simulink model "FullCardioLablModel"  (R2023b)
settings: Solver=FixedStepDiscrete  StartTime=0.0  StopTime=param_sim_time  FixedStep=1/fs  MaxStep=1/fs  RelTol=1e-3
undefined symbols (not defined in the file): analyses, fdesignblkfcn, fs, gcbh, param_tot_samples
libraries: dspstat3 x13, SCGAnalysis_SignalGenerationLib x2
(part 5 of 20)

== system FullCardioLablModel/ECG Preprocessing/Enabled ECG Preprocessing Subsystem/To Workspace: Processed ECG/Enabled To Workspace ECG Subsystem ==
  note: The subsystem is only enabled when it receives a (non-zero) signal
  In1 : Inport
  Enable : EnablePort
  To Workspace ECG : ToWorkspace  VariableName=out_ecg_preprocessing  SaveFormat=Structure  SampleTime=-1
  wires:
  In1/1 -> To Workspace ECG/1

== system FullCardioLablModel/SCG Analysis/Enabled SCG Analysis Subsystem/3D Anisotropy Characterization/Average Cycle Max Diameter//Volume Calculator ==
  in_r_pos : Inport
  in_scg_xyz : Inport  Port=2
  S1 Selector : Selector  NumberOfDimensions=2  InputPortWidth=3  IndexOptions=Index vector (dialog),Index vector (dialog)  Indices=[1:fs*0.2],[1 2 3]  OutputSizes=1,1
  SCG xyz Average Cycle : Subsystem
  Wrapped Average Cycle Max Diameter/Volume Calculator : MATLAB Function  TreatAsAtomicUnit=on
  out_average_cycle_max_diameter/volume : Outport
  wires:
  Wrapped Average Cycle Max Diameter/Volume Calculator/1(avg_cycle_max_diameter_over_volume) -> out_average_cycle_max_diameter/volume/1
  SCG xyz Average Cycle/1(out_scg_xyz_avgcycle) -> S1 Selector/1
  in_scg_xyz/1 -> SCG xyz Average Cycle/2(in_scg_xyz)
  in_r_pos/1 -> SCG xyz Average Cycle/1(in_ecg_r)
  S1 Selector/1 -> Wrapped Average Cycle Max Diameter/Volume Calculator/1(avg_s1_xyz)  "avg_scg_xyz_s1"

== system FullCardioLablModel/SCG Analysis/Enabled SCG Analysis Subsystem/3D Anisotropy Characterization/Average Cycle Max//Median Diameter Calculator ==
  in_r_pos : Inport
  in_scg_xyz : Inport  Port=2
  S1 Selector : Selector  NumberOfDimensions=2  InputPortWidth=3  IndexOptions=Index vector (dialog),Index vector (dialog)  Indices=[1:fs*0.2],[1 2 3]  OutputSizes=1,1
  SCG xyz Average Cycle : Subsystem
  Wrapped Average Cycle Max/Median Diameter Calculator : MATLAB Function  TreatAsAtomicUnit=on
  out_average_cycle_max/median_diameter : Outport
  wires:
  Wrapped Average Cycle Max/Median Diameter Calculator/1(avg_cycle_max_over_median_diameter) -> out_average_cycle_max/median_diameter/1
  SCG xyz Average Cycle/1(out_scg_xyz_avgcycle) -> S1 Selector/1
  in_scg_xyz/1 -> SCG xyz Average Cycle/2(in_scg_xyz)
  in_r_pos/1 -> SCG xyz Average Cycle/1(in_ecg_r)
  S1 Selector/1 -> Wrapped Average Cycle Max/Median Diameter Calculator/1(avg_s1_xyz)  "avg_scg_xyz_s1"

== system FullCardioLablModel/SCG Analysis/Enabled SCG Analysis Subsystem/3D Anisotropy Characterization/Average Cycle Max//Min Diameter Calculator ==
  in_r_pos : Inport
  in_scg_xyz : Inport  Port=2
  S1 Selector : Selector  NumberOfDimensions=2  InputPortWidth=3  IndexOptions=Index vector (dialog),Index vector (dialog)  Indices=[1:fs*0.2],[1 2 3]  OutputSizes=1,1
  SCG xyz Average Cycle : Subsystem
  Wrapped Average Cycle Max/Min Diameters Calculator : MATLAB Function  TreatAsAtomicUnit=on
  out_average_cycle_max/min_diameter : Outport
  wires:
  S1 Selector/1 -> Wrapped Average Cycle Max/Min Diameters Calculator/1(avg_s1_xyz)  "avg_scg_xyz_s1"
  in_r_pos/1 -> SCG xyz Average Cycle/1(in_ecg_r)
  in_scg_xyz/1 -> SCG xyz Average Cycle/2(in_scg_xyz)
  SCG xyz Average Cycle/1(out_scg_xyz_avgcycle) -> S1 Selector/1
  Wrapped Average Cycle Max/Min Diameters Calculator/1(avg_cycle_max_over_min_diameters) -> out_average_cycle_max/min_diameter/1

== system FullCardioLablModel/SCG Analysis/Enabled SCG Analysis Subsystem/3D Anisotropy Characterization/Average Max Diameter//Volume Calculator ==
  in_r_pos : Inport
  in_scg_xyz : Inport  Port=2
  Constant1 : Constant  Value=fs
  Wrapped Average Max Diameter/Volume Calculator : MATLAB Function  TreatAsAtomicUnit=on
  out_average_max_diameter/volume : Outport
  wires:
  Constant1/1 -> Wrapped Average Max Diameter/Volume Calculator/1(fs)
  Wrapped Average Max Diameter/Volume Calculator/1(avg_max_diameter_over_volume) -> out_average_max_diameter/volume/1
  in_scg_xyz/1 -> Wrapped Average Max Diameter/Volume Calculator/3(scg_xyz)
  in_r_pos/1 -> Wrapped Average Max Diameter/Volume Calculator/2(r_pos)

== system FullCardioLablModel/SCG Analysis/Enabled SCG Analysis Subsystem/3D Anisotropy Characterization/Average Max//Median Diameter Calculator ==
  in_r_pos : Inport
  in_scg_xyz : Inport  Port=2
  Constant1 : Constant  Value=fs
  Wrapped Average Max/Median Diameter Calculator : MATLAB Function  TreatAsAtomicUnit=on
  out_average_max/median_diameter : Outport
  wires:
  Constant1/1 -> Wrapped Average Max/Median Diameter Calculator/1(fs)
  Wrapped Average Max/Median Diameter Calculator/1(avg_max_over_median_diameter) -> out_average_max/median_diameter/1
  in_scg_xyz/1 -> Wrapped Average Max/Median Diameter Calculator/3(scg_xyz)
  in_r_pos/1 -> Wrapped Average Max/Median Diameter Calculator/2(r_pos)

== system FullCardioLablModel/SCG Analysis/Enabled SCG Analysis Subsystem/3D Anisotropy Characterization/Average Max//Min Diameter Calculator ==
  in_r_pos : Inport
  in_scg_xyz : Inport  Port=2
  Constant1 : Constant  Value=fs
  Wrapped Average Max/Min Diameters Calculator : MATLAB Function  TreatAsAtomicUnit=on
  out_average_max/min_diameter : Outport
  wires:
  in_r_pos/1 -> Wrapped Average Max/Min Diameters Calculator/2(r_pos)
  in_scg_xyz/1 -> Wrapped Average Max/Min Diameters Calculator/3(scg_xyz)
  Wrapped Average Max/Min Diameters Calculator/1(avg_max_over_min_diameters) -> out_average_max/min_diameter/1
  Constant1/1 -> Wrapped Average Max/Min Diameters Calculator/1(fs)

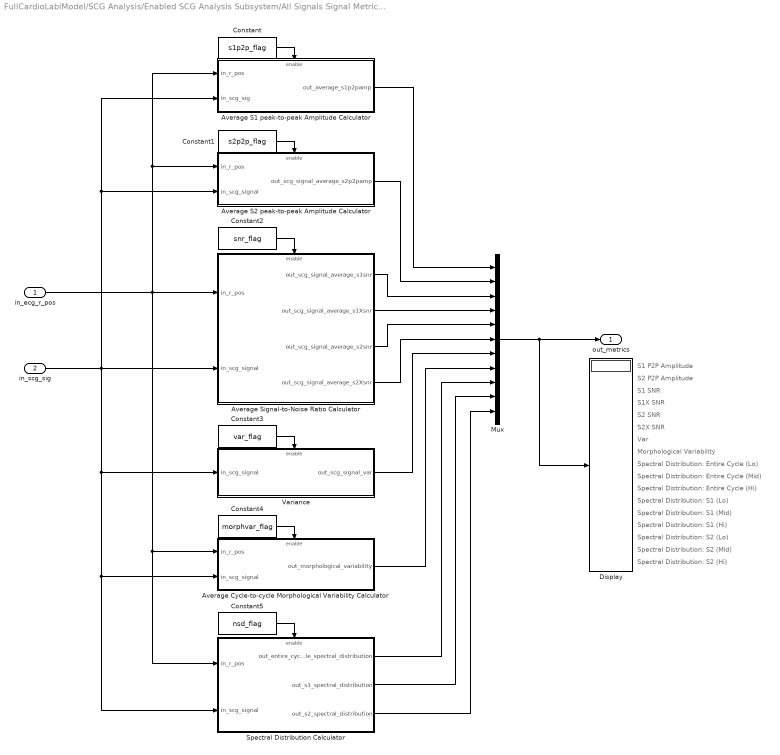
== system FullCardioLablModel/SCG Analysis/Enabled SCG Analysis Subsystem/All Signals Signal Metric Characterization/SCG 2D Mod Signal Metric Characterization ==
  note: S1 P2P Amplitude
  note: S2 P2P Amplitude
  note: S1 SNR
  note: S1X SNR
  note: S2 SNR
  note: S2X SNR
  note: Var
  note: Morphological Variability
  note: Spectral Distribution: Entire Cycle (Lo)
  note: Spectral Distribution: Entire Cycle (Mid)
  note: Spectral Distribution: Entire Cycle (Hi)
  note: Spectral Distribution: S1 (Lo)
  note: Spectral Distribution: S1 (Mid)
  note: Spectral Distribution: S1 (Hi)
  note: Spectral Distribution: S2 (Hi)
  note: Spectral Distribution: S2 (Lo)
  note: Spectral Distribution: S2 (Mid)
  in_ecg_r_pos : Inport
  in_scg_sig : Inport  Port=2
  Average Cycle-to-cycle Morphological Variability Calculator : Subsystem
  Average S1 peak-to-peak Amplitude Calculator : Subsystem
  Average S2 peak-to-peak Amplitude Calculator : Subsystem
  Average Signal-to-Noise Ratio Calculator : Subsystem  mask{s1snr_flag=on, s1xsnr_flag=on, s2snr_flag=on, s2xsnr_flag=on}
      mask prompts: s1snr_flag "S1 SnR"; s1xsnr_flag "S1X SnR (S2 complex is removed)"; s2snr_flag "S2 SnR"; s2xsnr_flag "S2X SnR (S1 complex is removed)"
      mask DialogControl DescGroupVar Prompt: Signal-to-Noise Ratio Characterization
      mask DialogControl DescTextVar Prompt: Block to quantify the signal to noise ratio of the S1 and S2 complexes. Two types of SnRs can be calculated: the normal SnR (which reflects the ease of performing an independent detection of that complex), and the exclusive SnR (which does not cosider the S2 or S1 complex in the case of the S1 and S2 SnRs, respectively).
      mask DialogControl Control2 Prompt: Choose which SnRs to compute:
  Constant : Constant  Value=s1p2p_flag
  Constant1 : Constant  Value=s2p2p_flag
  Constant2 : Constant  Value=snr_flag
  Constant3 : Constant  Value=var_flag
  Constant4 : Constant  Value=morphvar_flag
  Constant5 : Constant  Value=nsd_flag
  Display : Display
  Mux : Mux  Inputs=11
  Spectral Distribution Calculator : Subsystem  mask{entire_cycle=on, s1=on, s2=on, f_band_lo=[7.5 15], f_band_mid=[15 30], f_band_hi=[30 120]}
      mask prompts: entire_cycle "Entire Cycle"; s1 "S1 Complex"; s2 "S2 Complex"; f_band_lo "Frequency Band Low Limits (Hz)"; f_band_mid "Frequency Band Mid Limits (Hz)"; f_band_hi "Frequency Band Hi Limits (Hz)"
      mask DialogControl DescGroupVar Prompt: Spectral Distribution Calculator
      mask DialogControl DescTextVar Prompt: Block to calculate the (normalized) distrubtions of the power spectral densities of: the entire cycle, the S1 complex, and the S2 complex. First select which combination of spectral distrubtions to calculate. Then enter the frequency limits (in Hz) of the three contiguos bins that will define the spectral distribution.
      mask DialogControl ParameterGroupVar_copy Prompt: Spectral Distributions to Calculate
      mask DialogControl Control4 Prompt: Select which spectral distributions to calculate.
      mask DialogControl ParameterGroupVar Prompt: Bin Frequency Bands
      mask DialogControl Control2 Prompt: Enter the frequency limits (in Hz) inside square brackets for three contiguous bins (e.g. [5 10], [10 40], and [40 120]).
  Variance : Subsystem
  out_metrics : Outport
  wires:
  in_scg_sig/1 -> Average S2 peak-to-peak Amplitude Calculator/2(in_scg_signal), Average S1 peak-to-peak Amplitude Calculator/2(in_scg_sig), Average Signal-to-Noise Ratio Calculator/2(in_scg_signal), Spectral Distribution Calculator/2(in_scg_signal), Average Cycle-to-cycle Morphological Variability Calculator/2(in_scg_signal), Variance/1(in_scg_signal)
  Average S1 peak-to-peak Amplitude Calculator/1(out_average_s1p2pamp) -> Mux/1
  in_ecg_r_pos/1 -> Spectral Distribution Calculator/1(in_r_pos), Average Cycle-to-cycle Morphological Variability Calculator/1(in_r_pos), Average S2 peak-to-peak Amplitude Calculator/1(in_r_pos), Average S1 peak-to-peak Amplitude Calculator/1(in_r_pos), Average Signal-to-Noise Ratio Calculator/1(in_r_pos)
  Average Signal-to-Noise Ratio Calculator/2(out_scg_signal_average_s1Xsnr) -> Mux/4
  Average Signal-to-Noise Ratio Calculator/1(out_scg_signal_average_s1snr) -> Mux/3
  Average Signal-to-Noise Ratio Calculator/3(out_scg_signal_average_s2snr) -> Mux/5
  Average Signal-to-Noise Ratio Calculator/4(out_scg_signal_average_s2Xsnr) -> Mux/6
  Average S2 peak-to-peak Amplitude Calculator/1(out_scg_signal_average_s2p2pamp) -> Mux/2
  Average Cycle-to-cycle Morphological Variability Calculator/1(out_morphological_variability) -> Mux/8
  Spectral Distribution Calculator/1(out_entire_cycle_spectral_distribution) -> Mux/9
  Spectral Distribution Calculator/3(out_s2_spectral_distribution) -> Mux/11
  Spectral Distribution Calculator/2(out_s1_spectral_distribution) -> Mux/10
  Variance/1(out_scg_signal_var) -> Mux/7
  Constant/1 -> Average S1 peak-to-peak Amplitude Calculator/Enable
  Constant1/1 -> Average S2 peak-to-peak Amplitude Calculator/Enable
  Constant2/1 -> Average Signal-to-Noise Ratio Calculator/Enable
  Constant3/1 -> Variance/Enable
  Constant4/1 -> Average Cycle-to-cycle Morphological Variability Calculator/Enable
  Constant5/1 -> Spectral Distribution Calculator/Enable
  Mux/1 -> Display/1, out_metrics/1

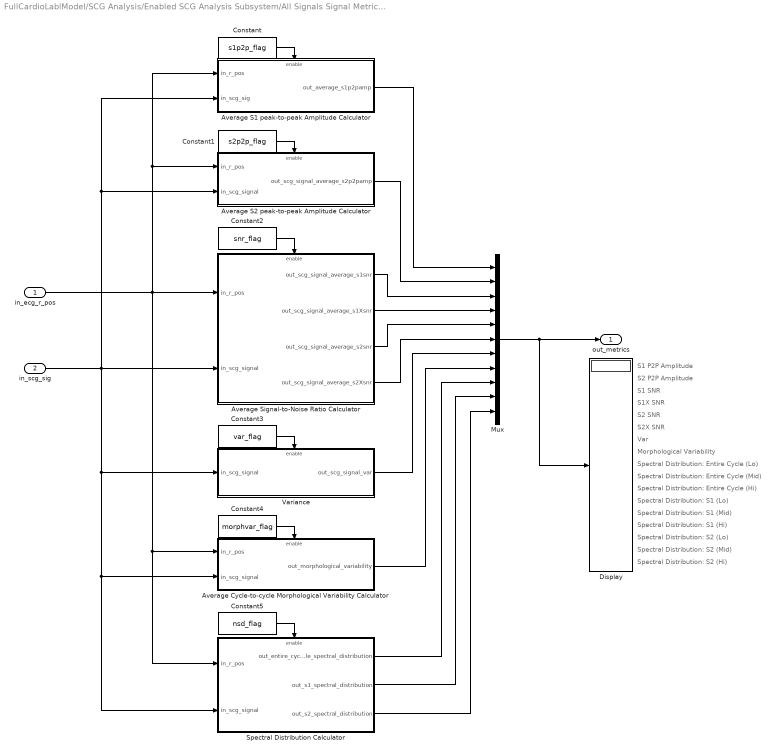
== system FullCardioLablModel/SCG Analysis/Enabled SCG Analysis Subsystem/All Signals Signal Metric Characterization/SCG 3D Mod Signal Metric Characterization ==
  note: Spectral Distribution: S2 (Mid)
  note: Spectral Distribution: S2 (Lo)
  note: Spectral Distribution: S2 (Hi)
  note: Spectral Distribution: S1 (Hi)
  note: Spectral Distribution: S1 (Mid)
  note: Spectral Distribution: S1 (Lo)
  note: Spectral Distribution: Entire Cycle (Hi)
  note: Spectral Distribution: Entire Cycle (Mid)
  note: Spectral Distribution: Entire Cycle (Lo)
  note: Morphological Variability
  note: Var
  note: S2X SNR
  note: S2 SNR
  note: S1X SNR
  note: S1 SNR
  note: S2 P2P Amplitude
  note: S1 P2P Amplitude
  in_ecg_r_pos : Inport
  in_scg_sig : Inport  Port=2
  Average Cycle-to-cycle Morphological Variability Calculator : Subsystem
  Average S1 peak-to-peak Amplitude Calculator : Subsystem
  Average S2 peak-to-peak Amplitude Calculator : Subsystem
  Average Signal-to-Noise Ratio Calculator : Subsystem  mask{s1snr_flag=on, s1xsnr_flag=on, s2snr_flag=on, s2xsnr_flag=on}
      mask prompts: s1snr_flag "S1 SnR"; s1xsnr_flag "S1X SnR (S2 complex is removed)"; s2snr_flag "S2 SnR"; s2xsnr_flag "S2X SnR (S1 complex is removed)"
      mask DialogControl DescGroupVar Prompt: Signal-to-Noise Ratio Characterization
      mask DialogControl DescTextVar Prompt: Block to quantify the signal to noise ratio of the S1 and S2 complexes. Two types of SnRs can be calculated: the normal SnR (which reflects the ease of performing an independent detection of that complex), and the exclusive SnR (which does not cosider the S2 or S1 complex in the case of the S1 and S2 SnRs, respectively).
      mask DialogControl Control2 Prompt: Choose which SnRs to compute:
  Constant : Constant  Value=s1p2p_flag
  Constant1 : Constant  Value=s2p2p_flag
  Constant2 : Constant  Value=snr_flag
  Constant3 : Constant  Value=var_flag
  Constant4 : Constant  Value=morphvar_flag
  Constant5 : Constant  Value=nsd_flag
  Display : Display
  Mux : Mux  Inputs=11
  Spectral Distribution Calculator : Subsystem  mask{entire_cycle=on, s1=on, s2=on, f_band_lo=[7.5 15], f_band_mid=[15 30], f_band_hi=[30 120]}
      mask prompts: entire_cycle "Entire Cycle"; s1 "S1 Complex"; s2 "S2 Complex"; f_band_lo "Frequency Band Low Limits (Hz)"; f_band_mid "Frequency Band Mid Limits (Hz)"; f_band_hi "Frequency Band Hi Limits (Hz)"
      mask DialogControl DescGroupVar Prompt: Spectral Distribution Calculator
      mask DialogControl DescTextVar Prompt: Block to calculate the (normalized) distrubtions of the power spectral densities of: the entire cycle, the S1 complex, and the S2 complex. First select which combination of spectral distrubtions to calculate. Then enter the frequency limits (in Hz) of the three contiguos bins that will define the spectral distribution.
      mask DialogControl ParameterGroupVar_copy Prompt: Spectral Distributions to Calculate
      mask DialogControl Control4 Prompt: Select which spectral distributions to calculate.
      mask DialogControl ParameterGroupVar Prompt: Bin Frequency Bands
      mask DialogControl Control2 Prompt: Enter the frequency limits (in Hz) inside square brackets for three contiguous bins (e.g. [5 10], [10 40], and [40 120]).
  Variance : Subsystem
  out_metrics : Outport
  wires:
  Mux/1 -> out_metrics/1, Display/1
  Constant5/1 -> Spectral Distribution Calculator/Enable
  Constant4/1 -> Average Cycle-to-cycle Morphological Variability Calculator/Enable
  Constant3/1 -> Variance/Enable
  Constant2/1 -> Average Signal-to-Noise Ratio Calculator/Enable
  Constant1/1 -> Average S2 peak-to-peak Amplitude Calculator/Enable
  Constant/1 -> Average S1 peak-to-peak Amplitude Calculator/Enable
  Variance/1(out_scg_signal_var) -> Mux/7
  Spectral Distribution Calculator/2(out_s1_spectral_distribution) -> Mux/10
  Spectral Distribution Calculator/3(out_s2_spectral_distribution) -> Mux/11
  Spectral Distribution Calculator/1(out_entire_cycle_spectral_distribution) -> Mux/9
  Average Cycle-to-cycle Morphological Variability Calculator/1(out_morphological_variability) -> Mux/8
  Average S2 peak-to-peak Amplitude Calculator/1(out_scg_signal_average_s2p2pamp) -> Mux/2
  Average Signal-to-Noise Ratio Calculator/4(out_scg_signal_average_s2Xsnr) -> Mux/6
  Average Signal-to-Noise Ratio Calculator/3(out_scg_signal_average_s2snr) -> Mux/5
  Average Signal-to-Noise Ratio Calculator/1(out_scg_signal_average_s1snr) -> Mux/3
  Average Signal-to-Noise Ratio Calculator/2(out_scg_signal_average_s1Xsnr) -> Mux/4
  in_ecg_r_pos/1 -> Average Signal-to-Noise Ratio Calculator/1(in_r_pos), Average S1 peak-to-peak Amplitude Calculator/1(in_r_pos), Average S2 peak-to-peak Amplitude Calculator/1(in_r_pos), Average Cycle-to-cycle Morphological Variability Calculator/1(in_r_pos), Spectral Distribution Calculator/1(in_r_pos)
  Average S1 peak-to-peak Amplitude Calculator/1(out_average_s1p2pamp) -> Mux/1
  in_scg_sig/1 -> Average S1 peak-to-peak Amplitude Calculator/2(in_scg_sig), Average S2 peak-to-peak Amplitude Calculator/2(in_scg_signal), Average Signal-to-Noise Ratio Calculator/2(in_scg_signal), Variance/1(in_scg_signal), Average Cycle-to-cycle Morphological Variability Calculator/2(in_scg_signal), Spectral Distribution Calculator/2(in_scg_signal)

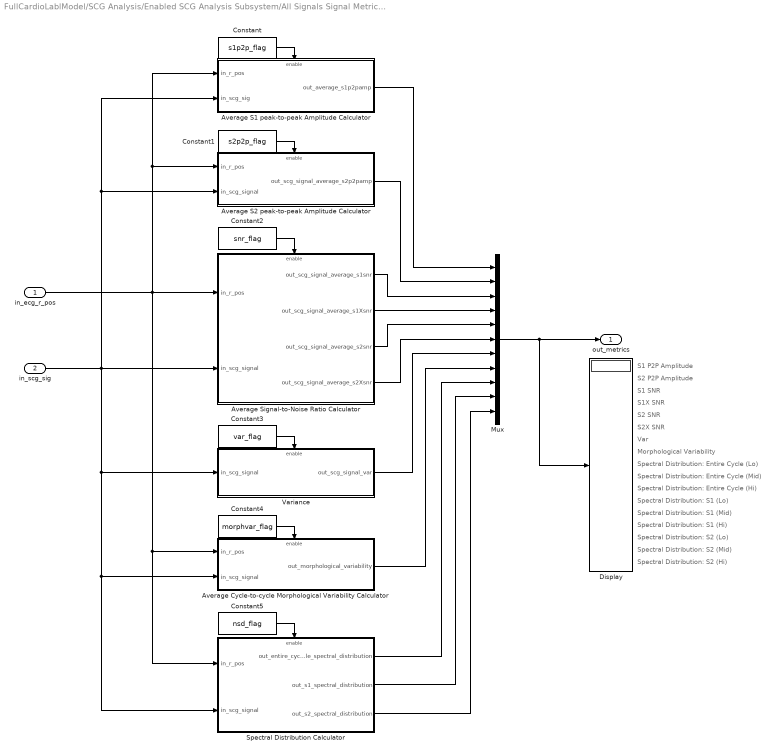
== system FullCardioLablModel/SCG Analysis/Enabled SCG Analysis Subsystem/All Signals Signal Metric Characterization/SCG 3DMaxS2p2pProjection Signal Metric Characterization ==
  note: Spectral Distribution: S2 (Mid)
  note: Spectral Distribution: S2 (Lo)
  note: Spectral Distribution: S2 (Hi)
  note: Spectral Distribution: S1 (Hi)
  note: Spectral Distribution: S1 (Mid)
  note: Spectral Distribution: S1 (Lo)
  note: Spectral Distribution: Entire Cycle (Hi)
  note: Spectral Distribution: Entire Cycle (Mid)
  note: Spectral Distribution: Entire Cycle (Lo)
  note: Morphological Variability
  note: Var
  note: S2X SNR
  note: S2 SNR
  note: S1X SNR
  note: S1 SNR
  note: S2 P2P Amplitude
  note: S1 P2P Amplitude
  in_ecg_r_pos : Inport
  in_scg_sig : Inport  Port=2
  Average Cycle-to-cycle Morphological Variability Calculator : Subsystem
  Average S1 peak-to-peak Amplitude Calculator : Subsystem
  Average S2 peak-to-peak Amplitude Calculator : Subsystem
  Average Signal-to-Noise Ratio Calculator : Subsystem  mask{s1snr_flag=on, s1xsnr_flag=on, s2snr_flag=on, s2xsnr_flag=on}
      mask prompts: s1snr_flag "S1 SnR"; s1xsnr_flag "S1X SnR (S2 complex is removed)"; s2snr_flag "S2 SnR"; s2xsnr_flag "S2X SnR (S1 complex is removed)"
      mask DialogControl DescGroupVar Prompt: Signal-to-Noise Ratio Characterization
      mask DialogControl DescTextVar Prompt: Block to quantify the signal to noise ratio of the S1 and S2 complexes. Two types of SnRs can be calculated: the normal SnR (which reflects the ease of performing an independent detection of that complex), and the exclusive SnR (which does not cosider the S2 or S1 complex in the case of the S1 and S2 SnRs, respectively).
      mask DialogControl Control2 Prompt: Choose which SnRs to compute:
  Constant : Constant  Value=s1p2p_flag
  Constant1 : Constant  Value=s2p2p_flag
  Constant2 : Constant  Value=snr_flag
  Constant3 : Constant  Value=var_flag
  Constant4 : Constant  Value=morphvar_flag
  Constant5 : Constant  Value=nsd_flag
  Display : Display
  Mux : Mux  Inputs=11
  Spectral Distribution Calculator : Subsystem  mask{entire_cycle=on, s1=on, s2=on, f_band_lo=[7.5 15], f_band_mid=[15 30], f_band_hi=[30 120]}
      mask prompts: entire_cycle "Entire Cycle"; s1 "S1 Complex"; s2 "S2 Complex"; f_band_lo "Frequency Band Low Limits (Hz)"; f_band_mid "Frequency Band Mid Limits (Hz)"; f_band_hi "Frequency Band Hi Limits (Hz)"
      mask DialogControl DescGroupVar Prompt: Spectral Distribution Calculator
      mask DialogControl DescTextVar Prompt: Block to calculate the (normalized) distrubtions of the power spectral densities of: the entire cycle, the S1 complex, and the S2 complex. First select which combination of spectral distrubtions to calculate. Then enter the frequency limits (in Hz) of the three contiguos bins that will define the spectral distribution.
      mask DialogControl ParameterGroupVar_copy Prompt: Spectral Distributions to Calculate
      mask DialogControl Control4 Prompt: Select which spectral distributions to calculate.
      mask DialogControl ParameterGroupVar Prompt: Bin Frequency Bands
      mask DialogControl Control2 Prompt: Enter the frequency limits (in Hz) inside square brackets for three contiguous bins (e.g. [5 10], [10 40], and [40 120]).
  Variance : Subsystem
  out_metrics : Outport
  wires:
  Mux/1 -> out_metrics/1, Display/1
  Constant5/1 -> Spectral Distribution Calculator/Enable
  Constant4/1 -> Average Cycle-to-cycle Morphological Variability Calculator/Enable
  Constant3/1 -> Variance/Enable
  Constant2/1 -> Average Signal-to-Noise Ratio Calculator/Enable
  Constant1/1 -> Average S2 peak-to-peak Amplitude Calculator/Enable
  Constant/1 -> Average S1 peak-to-peak Amplitude Calculator/Enable
  Variance/1(out_scg_signal_var) -> Mux/7
  Spectral Distribution Calculator/2(out_s1_spectral_distribution) -> Mux/10
  Spectral Distribution Calculator/3(out_s2_spectral_distribution) -> Mux/11
  Spectral Distribution Calculator/1(out_entire_cycle_spectral_distribution) -> Mux/9
  Average Cycle-to-cycle Morphological Variability Calculator/1(out_morphological_variability) -> Mux/8
  Average S2 peak-to-peak Amplitude Calculator/1(out_scg_signal_average_s2p2pamp) -> Mux/2
  Average Signal-to-Noise Ratio Calculator/4(out_scg_signal_average_s2Xsnr) -> Mux/6
  Average Signal-to-Noise Ratio Calculator/3(out_scg_signal_average_s2snr) -> Mux/5
  Average Signal-to-Noise Ratio Calculator/1(out_scg_signal_average_s1snr) -> Mux/3
  Average Signal-to-Noise Ratio Calculator/2(out_scg_signal_average_s1Xsnr) -> Mux/4
  in_ecg_r_pos/1 -> Average Signal-to-Noise Ratio Calculator/1(in_r_pos), Average S1 peak-to-peak Amplitude Calculator/1(in_r_pos), Average S2 peak-to-peak Amplitude Calculator/1(in_r_pos), Average Cycle-to-cycle Morphological Variability Calculator/1(in_r_pos), Spectral Distribution Calculator/1(in_r_pos)
  Average S1 peak-to-peak Amplitude Calculator/1(out_average_s1p2pamp) -> Mux/1
  in_scg_sig/1 -> Average S1 peak-to-peak Amplitude Calculator/2(in_scg_sig), Average S2 peak-to-peak Amplitude Calculator/2(in_scg_signal), Average Signal-to-Noise Ratio Calculator/2(in_scg_signal), Variance/1(in_scg_signal), Average Cycle-to-cycle Morphological Variability Calculator/2(in_scg_signal), Spectral Distribution Calculator/2(in_scg_signal)

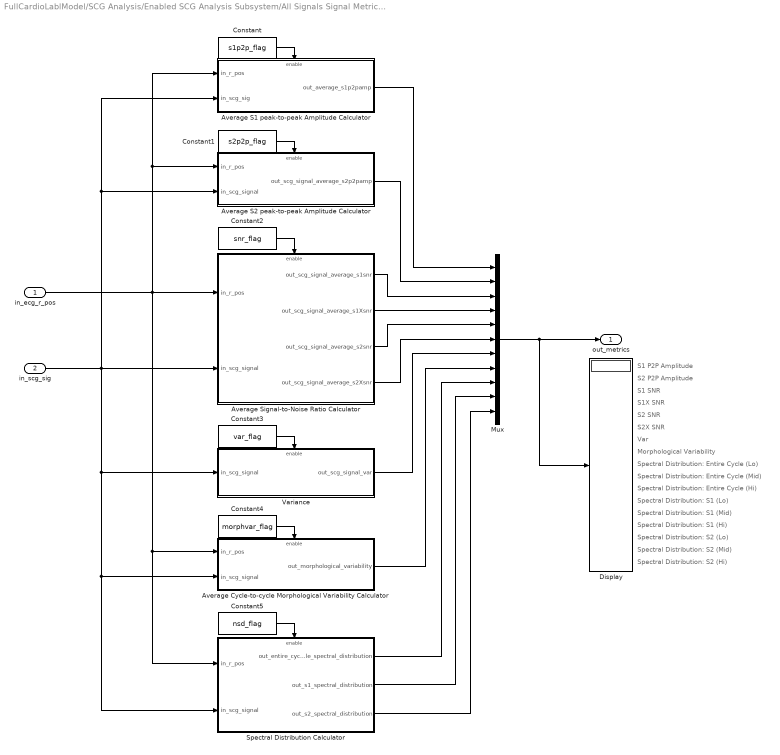
== system FullCardioLablModel/SCG Analysis/Enabled SCG Analysis Subsystem/All Signals Signal Metric Characterization/SCG 3DMinS2p2pProjection Signal Metric Characterization ==
  note: S1 P2P Amplitude
  note: S2 P2P Amplitude
  note: S1 SNR
  note: S1X SNR
  note: S2 SNR
  note: S2X SNR
  note: Var
  note: Morphological Variability
  note: Spectral Distribution: Entire Cycle (Lo)
  note: Spectral Distribution: Entire Cycle (Mid)
  note: Spectral Distribution: Entire Cycle (Hi)
  note: Spectral Distribution: S1 (Lo)
  note: Spectral Distribution: S1 (Mid)
  note: Spectral Distribution: S1 (Hi)
  note: Spectral Distribution: S2 (Hi)
  note: Spectral Distribution: S2 (Lo)
  note: Spectral Distribution: S2 (Mid)
  in_ecg_r_pos : Inport
  in_scg_sig : Inport  Port=2
  Average Cycle-to-cycle Morphological Variability Calculator : Subsystem
  Average S1 peak-to-peak Amplitude Calculator : Subsystem
  Average S2 peak-to-peak Amplitude Calculator : Subsystem
  Average Signal-to-Noise Ratio Calculator : Subsystem  mask{s1snr_flag=on, s1xsnr_flag=on, s2snr_flag=on, s2xsnr_flag=on}
      mask prompts: s1snr_flag "S1 SnR"; s1xsnr_flag "S1X SnR (S2 complex is removed)"; s2snr_flag "S2 SnR"; s2xsnr_flag "S2X SnR (S1 complex is removed)"
      mask DialogControl DescGroupVar Prompt: Signal-to-Noise Ratio Characterization
      mask DialogControl DescTextVar Prompt: Block to quantify the signal to noise ratio of the S1 and S2 complexes. Two types of SnRs can be calculated: the normal SnR (which reflects the ease of performing an independent detection of that complex), and the exclusive SnR (which does not cosider the S2 or S1 complex in the case of the S1 and S2 SnRs, respectively).
      mask DialogControl Control2 Prompt: Choose which SnRs to compute:
  Constant : Constant  Value=s1p2p_flag
  Constant1 : Constant  Value=s2p2p_flag
  Constant2 : Constant  Value=snr_flag
  Constant3 : Constant  Value=var_flag
  Constant4 : Constant  Value=morphvar_flag
  Constant5 : Constant  Value=nsd_flag
  Display : Display
  Mux : Mux  Inputs=11
  Spectral Distribution Calculator : Subsystem  mask{entire_cycle=on, s1=on, s2=on, f_band_lo=[7.5 15], f_band_mid=[15 30], f_band_hi=[30 120]}
      mask prompts: entire_cycle "Entire Cycle"; s1 "S1 Complex"; s2 "S2 Complex"; f_band_lo "Frequency Band Low Limits (Hz)"; f_band_mid "Frequency Band Mid Limits (Hz)"; f_band_hi "Frequency Band Hi Limits (Hz)"
      mask DialogControl DescGroupVar Prompt: Spectral Distribution Calculator
      mask DialogControl DescTextVar Prompt: Block to calculate the (normalized) distrubtions of the power spectral densities of: the entire cycle, the S1 complex, and the S2 complex. First select which combination of spectral distrubtions to calculate. Then enter the frequency limits (in Hz) of the three contiguos bins that will define the spectral distribution.
      mask DialogControl ParameterGroupVar_copy Prompt: Spectral Distributions to Calculate
      mask DialogControl Control4 Prompt: Select which spectral distributions to calculate.
      mask DialogControl ParameterGroupVar Prompt: Bin Frequency Bands
      mask DialogControl Control2 Prompt: Enter the frequency limits (in Hz) inside square brackets for three contiguous bins (e.g. [5 10], [10 40], and [40 120]).
  Variance : Subsystem
  out_metrics : Outport
  wires:
  in_scg_sig/1 -> Average S2 peak-to-peak Amplitude Calculator/2(in_scg_signal), Average S1 peak-to-peak Amplitude Calculator/2(in_scg_sig), Spectral Distribution Calculator/2(in_scg_signal), Average Cycle-to-cycle Morphological Variability Calculator/2(in_scg_signal), Variance/1(in_scg_signal), Average Signal-to-Noise Ratio Calculator/2(in_scg_signal)
  Average S1 peak-to-peak Amplitude Calculator/1(out_average_s1p2pamp) -> Mux/1
  in_ecg_r_pos/1 -> Spectral Distribution Calculator/1(in_r_pos), Average Cycle-to-cycle Morphological Variability Calculator/1(in_r_pos), Average S2 peak-to-peak Amplitude Calculator/1(in_r_pos), Average S1 peak-to-peak Amplitude Calculator/1(in_r_pos), Average Signal-to-Noise Ratio Calculator/1(in_r_pos)
  Average Signal-to-Noise Ratio Calculator/2(out_scg_signal_average_s1Xsnr) -> Mux/4
  Average Signal-to-Noise Ratio Calculator/1(out_scg_signal_average_s1snr) -> Mux/3
  Average Signal-to-Noise Ratio Calculator/3(out_scg_signal_average_s2snr) -> Mux/5
  Average Signal-to-Noise Ratio Calculator/4(out_scg_signal_average_s2Xsnr) -> Mux/6
  Average S2 peak-to-peak Amplitude Calculator/1(out_scg_signal_average_s2p2pamp) -> Mux/2
  Average Cycle-to-cycle Morphological Variability Calculator/1(out_morphological_variability) -> Mux/8
  Spectral Distribution Calculator/1(out_entire_cycle_spectral_distribution) -> Mux/9
  Spectral Distribution Calculator/3(out_s2_spectral_distribution) -> Mux/11
  Spectral Distribution Calculator/2(out_s1_spectral_distribution) -> Mux/10
  Variance/1(out_scg_signal_var) -> Mux/7
  Constant/1 -> Average S1 peak-to-peak Amplitude Calculator/Enable
  Constant1/1 -> Average S2 peak-to-peak Amplitude Calculator/Enable
  Constant2/1 -> Average Signal-to-Noise Ratio Calculator/Enable
  Constant3/1 -> Variance/Enable
  Constant4/1 -> Average Cycle-to-cycle Morphological Variability Calculator/Enable
  Constant5/1 -> Spectral Distribution Calculator/Enable
  Mux/1 -> Display/1, out_metrics/1

== system FullCardioLablModel/SCG Analysis/Enabled SCG Analysis Subsystem/All Signals Signal Metric Characterization/SCG S2 3DAntiMechAxis Signal Metric Characterization ==
  note: S1 P2P Amplitude
  note: S2 P2P Amplitude
  note: S1 SNR
  note: S1X SNR
  note: S2 SNR
  note: S2X SNR
  note: Var
  note: Morphological Variability
  note: Spectral Distribution: Entire Cycle (Lo)
  note: Spectral Distribution: Entire Cycle (Mid)
  note: Spectral Distribution: Entire Cycle (Hi)
  note: Spectral Distribution: S1 (Lo)
  note: Spectral Distribution: S1 (Mid)
  note: Spectral Distribution: S1 (Hi)
  note: Spectral Distribution: S2 (Hi)
  note: Spectral Distribution: S2 (Lo)
  note: Spectral Distribution: S2 (Mid)
  in_ecg_r_pos : Inport
  in_scg_sig : Inport  Port=2
  Average Cycle-to-cycle Morphological Variability Calculator : Subsystem
  Average S1 peak-to-peak Amplitude Calculator : Subsystem
  Average S2 peak-to-peak Amplitude Calculator : Subsystem
  Average Signal-to-Noise Ratio Calculator : Subsystem  mask{s1snr_flag=on, s1xsnr_flag=on, s2snr_flag=on, s2xsnr_flag=on}
      mask prompts: s1snr_flag "S1 SnR"; s1xsnr_flag "S1X SnR (S2 complex is removed)"; s2snr_flag "S2 SnR"; s2xsnr_flag "S2X SnR (S1 complex is removed)"
      mask DialogControl DescGroupVar Prompt: Signal-to-Noise Ratio Characterization
      mask DialogControl DescTextVar Prompt: Block to quantify the signal to noise ratio of the S1 and S2 complexes. Two types of SnRs can be calculated: the normal SnR (which reflects the ease of performing an independent detection of that complex), and the exclusive SnR (which does not cosider the S2 or S1 complex in the case of the S1 and S2 SnRs, respectively).
      mask DialogControl Control2 Prompt: Choose which SnRs to compute:
  Constant : Constant  Value=s1p2p_flag
  Constant1 : Constant  Value=s2p2p_flag
  Constant2 : Constant  Value=snr_flag
  Constant3 : Constant  Value=var_flag
  Constant4 : Constant  Value=morphvar_flag
  Constant5 : Constant  Value=nsd_flag
  Display : Display
  Mux : Mux  Inputs=11
  Spectral Distribution Calculator : Subsystem  mask{entire_cycle=on, s1=on, s2=on, f_band_lo=[7.5 15], f_band_mid=[15 30], f_band_hi=[30 120]}
      mask prompts: entire_cycle "Entire Cycle"; s1 "S1 Complex"; s2 "S2 Complex"; f_band_lo "Frequency Band Low Limits (Hz)"; f_band_mid "Frequency Band Mid Limits (Hz)"; f_band_hi "Frequency Band Hi Limits (Hz)"
      mask DialogControl DescGroupVar Prompt: Spectral Distribution Calculator
      mask DialogControl DescTextVar Prompt: Block to calculate the (normalized) distrubtions of the power spectral densities of: the entire cycle, the S1 complex, and the S2 complex. First select which combination of spectral distrubtions to calculate. Then enter the frequency limits (in Hz) of the three contiguos bins that will define the spectral distribution.
      mask DialogControl ParameterGroupVar_copy Prompt: Spectral Distributions to Calculate
      mask DialogControl Control4 Prompt: Select which spectral distributions to calculate.
      mask DialogControl ParameterGroupVar Prompt: Bin Frequency Bands
      mask DialogControl Control2 Prompt: Enter the frequency limits (in Hz) inside square brackets for three contiguous bins (e.g. [5 10], [10 40], and [40 120]).
  Variance : Subsystem
  out_metrics : Outport
  wires:
  in_scg_sig/1 -> Average S2 peak-to-peak Amplitude Calculator/2(in_scg_signal), Average S1 peak-to-peak Amplitude Calculator/2(in_scg_sig), Spectral Distribution Calculator/2(in_scg_signal), Average Cycle-to-cycle Morphological Variability Calculator/2(in_scg_signal), Variance/1(in_scg_signal), Average Signal-to-Noise Ratio Calculator/2(in_scg_signal)
  Average S1 peak-to-peak Amplitude Calculator/1(out_average_s1p2pamp) -> Mux/1
  in_ecg_r_pos/1 -> Spectral Distribution Calculator/1(in_r_pos), Average Cycle-to-cycle Morphological Variability Calculator/1(in_r_pos), Average S2 peak-to-peak Amplitude Calculator/1(in_r_pos), Average S1 peak-to-peak Amplitude Calculator/1(in_r_pos), Average Signal-to-Noise Ratio Calculator/1(in_r_pos)
  Average Signal-to-Noise Ratio Calculator/2(out_scg_signal_average_s1Xsnr) -> Mux/4
  Average Signal-to-Noise Ratio Calculator/1(out_scg_signal_average_s1snr) -> Mux/3
  Average Signal-to-Noise Ratio Calculator/3(out_scg_signal_average_s2snr) -> Mux/5
  Average Signal-to-Noise Ratio Calculator/4(out_scg_signal_average_s2Xsnr) -> Mux/6
  Average S2 peak-to-peak Amplitude Calculator/1(out_scg_signal_average_s2p2pamp) -> Mux/2
  Average Cycle-to-cycle Morphological Variability Calculator/1(out_morphological_variability) -> Mux/8
  Spectral Distribution Calculator/1(out_entire_cycle_spectral_distribution) -> Mux/9
  Spectral Distribution Calculator/3(out_s2_spectral_distribution) -> Mux/11
  Spectral Distribution Calculator/2(out_s1_spectral_distribution) -> Mux/10
  Variance/1(out_scg_signal_var) -> Mux/7
  Constant/1 -> Average S1 peak-to-peak Amplitude Calculator/Enable
  Constant1/1 -> Average S2 peak-to-peak Amplitude Calculator/Enable
  Constant2/1 -> Average Signal-to-Noise Ratio Calculator/Enable
  Constant3/1 -> Variance/Enable
  Constant4/1 -> Average Cycle-to-cycle Morphological Variability Calculator/Enable
  Constant5/1 -> Spectral Distribution Calculator/Enable
  Mux/1 -> Display/1, out_metrics/1

== system FullCardioLablModel/SCG Analysis/Enabled SCG Analysis Subsystem/All Signals Signal Metric Characterization/SCG S2 3DMechAxis Signal Metric Characterization ==
  note: Spectral Distribution: S2 (Mid)
  note: Spectral Distribution: S2 (Lo)
  note: Spectral Distribution: S2 (Hi)
  note: Spectral Distribution: S1 (Hi)
  note: Spectral Distribution: S1 (Mid)
  note: Spectral Distribution: S1 (Lo)
  note: Spectral Distribution: Entire Cycle (Hi)
  note: Spectral Distribution: Entire Cycle (Mid)
  note: Spectral Distribution: Entire Cycle (Lo)
  note: Morphological Variability
  note: Var
  note: S2X SNR
  note: S2 SNR
  note: S1X SNR
  note: S1 SNR
  note: S2 P2P Amplitude
  note: S1 P2P Amplitude
  in_ecg_r_pos : Inport
  in_scg_sig : Inport  Port=2
  Average Cycle-to-cycle Morphological Variability Calculator : Subsystem
  Average S1 peak-to-peak Amplitude Calculator : Subsystem
  Average S2 peak-to-peak Amplitude Calculator : Subsystem
  Average Signal-to-Noise Ratio Calculator : Subsystem  mask{s1snr_flag=on, s1xsnr_flag=on, s2snr_flag=on, s2xsnr_flag=on}
      mask prompts: s1snr_flag "S1 SnR"; s1xsnr_flag "S1X SnR (S2 complex is removed)"; s2snr_flag "S2 SnR"; s2xsnr_flag "S2X SnR (S1 complex is removed)"
      mask DialogControl DescGroupVar Prompt: Signal-to-Noise Ratio Characterization
      mask DialogControl DescTextVar Prompt: Block to quantify the signal to noise ratio of the S1 and S2 complexes. Two types of SnRs can be calculated: the normal SnR (which reflects the ease of performing an independent detection of that complex), and the exclusive SnR (which does not cosider the S2 or S1 complex in the case of the S1 and S2 SnRs, respectively).
      mask DialogControl Control2 Prompt: Choose which SnRs to compute:
  Constant : Constant  Value=s1p2p_flag
  Constant1 : Constant  Value=s2p2p_flag
  Constant2 : Constant  Value=snr_flag
  Constant3 : Constant  Value=var_flag
  Constant4 : Constant  Value=morphvar_flag
  Constant5 : Constant  Value=nsd_flag
  Display : Display
  Mux : Mux  Inputs=11
  Spectral Distribution Calculator : Subsystem  mask{entire_cycle=on, s1=on, s2=on, f_band_lo=[7.5 15], f_band_mid=[15 30], f_band_hi=[30 120]}
      mask prompts: entire_cycle "Entire Cycle"; s1 "S1 Complex"; s2 "S2 Complex"; f_band_lo "Frequency Band Low Limits (Hz)"; f_band_mid "Frequency Band Mid Limits (Hz)"; f_band_hi "Frequency Band Hi Limits (Hz)"
      mask DialogControl DescGroupVar Prompt: Spectral Distribution Calculator
      mask DialogControl DescTextVar Prompt: Block to calculate the (normalized) distrubtions of the power spectral densities of: the entire cycle, the S1 complex, and the S2 complex. First select which combination of spectral distrubtions to calculate. Then enter the frequency limits (in Hz) of the three contiguos bins that will define the spectral distribution.
      mask DialogControl ParameterGroupVar_copy Prompt: Spectral Distributions to Calculate
      mask DialogControl Control4 Prompt: Select which spectral distributions to calculate.
      mask DialogControl ParameterGroupVar Prompt: Bin Frequency Bands
      mask DialogControl Control2 Prompt: Enter the frequency limits (in Hz) inside square brackets for three contiguous bins (e.g. [5 10], [10 40], and [40 120]).
  Variance : Subsystem
  out_metrics : Outport
  wires:
  Mux/1 -> out_metrics/1, Display/1
  Constant5/1 -> Spectral Distribution Calculator/Enable
  Constant4/1 -> Average Cycle-to-cycle Morphological Variability Calculator/Enable
  Constant3/1 -> Variance/Enable
  Constant2/1 -> Average Signal-to-Noise Ratio Calculator/Enable
  Constant1/1 -> Average S2 peak-to-peak Amplitude Calculator/Enable
  Constant/1 -> Average S1 peak-to-peak Amplitude Calculator/Enable
  Variance/1(out_scg_signal_var) -> Mux/7
  Spectral Distribution Calculator/2(out_s1_spectral_distribution) -> Mux/10
  Spectral Distribution Calculator/3(out_s2_spectral_distribution) -> Mux/11
  Spectral Distribution Calculator/1(out_entire_cycle_spectral_distribution) -> Mux/9
  Average Cycle-to-cycle Morphological Variability Calculator/1(out_morphological_variability) -> Mux/8
  Average S2 peak-to-peak Amplitude Calculator/1(out_scg_signal_average_s2p2pamp) -> Mux/2
  Average Signal-to-Noise Ratio Calculator/4(out_scg_signal_average_s2Xsnr) -> Mux/6
  Average Signal-to-Noise Ratio Calculator/3(out_scg_signal_average_s2snr) -> Mux/5
  Average Signal-to-Noise Ratio Calculator/1(out_scg_signal_average_s1snr) -> Mux/3
  Average Signal-to-Noise Ratio Calculator/2(out_scg_signal_average_s1Xsnr) -> Mux/4
  in_ecg_r_pos/1 -> Average Signal-to-Noise Ratio Calculator/1(in_r_pos), Average S1 peak-to-peak Amplitude Calculator/1(in_r_pos), Average S2 peak-to-peak Amplitude Calculator/1(in_r_pos), Average Cycle-to-cycle Morphological Variability Calculator/1(in_r_pos), Spectral Distribution Calculator/1(in_r_pos)
  Average S1 peak-to-peak Amplitude Calculator/1(out_average_s1p2pamp) -> Mux/1
  in_scg_sig/1 -> Average Signal-to-Noise Ratio Calculator/2(in_scg_signal), Variance/1(in_scg_signal), Average Cycle-to-cycle Morphological Variability Calculator/2(in_scg_signal), Spectral Distribution Calculator/2(in_scg_signal), Average S1 peak-to-peak Amplitude Calculator/2(in_scg_sig), Average S2 peak-to-peak Amplitude Calculator/2(in_scg_signal)

== system FullCardioLablModel/SCG Analysis/Enabled SCG Analysis Subsystem/All Signals Signal Metric Characterization/SCG Systolic 3DAntiMechAxis Signal Metric Characterization ==
  note: S1 P2P Amplitude
  note: S2 P2P Amplitude
  note: S1 SNR
  note: S1X SNR
  note: S2 SNR
  note: S2X SNR
  note: Var
  note: Morphological Variability
  note: Spectral Distribution: Entire Cycle (Lo)
  note: Spectral Distribution: Entire Cycle (Mid)
  note: Spectral Distribution: Entire Cycle (Hi)
  note: Spectral Distribution: S1 (Lo)
  note: Spectral Distribution: S1 (Mid)
  note: Spectral Distribution: S1 (Hi)
  note: Spectral Distribution: S2 (Hi)
  note: Spectral Distribution: S2 (Lo)
  note: Spectral Distribution: S2 (Mid)
  in_ecg_r_pos : Inport
  in_scg_sig : Inport  Port=2
  Average Cycle-to-cycle Morphological Variability Calculator : Subsystem
  Average S1 peak-to-peak Amplitude Calculator : Subsystem
  Average S2 peak-to-peak Amplitude Calculator : Subsystem
  Average Signal-to-Noise Ratio Calculator : Subsystem  mask{s1snr_flag=on, s1xsnr_flag=on, s2snr_flag=on, s2xsnr_flag=on}
      mask prompts: s1snr_flag "S1 SnR"; s1xsnr_flag "S1X SnR (S2 complex is removed)"; s2snr_flag "S2 SnR"; s2xsnr_flag "S2X SnR (S1 complex is removed)"
      mask DialogControl DescGroupVar Prompt: Signal-to-Noise Ratio Characterization
      mask DialogControl DescTextVar Prompt: Block to quantify the signal to noise ratio of the S1 and S2 complexes. Two types of SnRs can be calculated: the normal SnR (which reflects the ease of performing an independent detection of that complex), and the exclusive SnR (which does not cosider the S2 or S1 complex in the case of the S1 and S2 SnRs, respectively).
      mask DialogControl Control2 Prompt: Choose which SnRs to compute:
  Constant : Constant  Value=s1p2p_flag
  Constant1 : Constant  Value=s2p2p_flag
  Constant2 : Constant  Value=snr_flag
  Constant3 : Constant  Value=var_flag
  Constant4 : Constant  Value=morphvar_flag
  Constant5 : Constant  Value=nsd_flag
  Display : Display
  Mux : Mux  Inputs=11
  Spectral Distribution Calculator : Subsystem  mask{entire_cycle=on, s1=on, s2=on, f_band_lo=[7.5 15], f_band_mid=[15 30], f_band_hi=[30 120]}
      mask prompts: entire_cycle "Entire Cycle"; s1 "S1 Complex"; s2 "S2 Complex"; f_band_lo "Frequency Band Low Limits (Hz)"; f_band_mid "Frequency Band Mid Limits (Hz)"; f_band_hi "Frequency Band Hi Limits (Hz)"
      mask DialogControl DescGroupVar Prompt: Spectral Distribution Calculator
      mask DialogControl DescTextVar Prompt: Block to calculate the (normalized) distrubtions of the power spectral densities of: the entire cycle, the S1 complex, and the S2 complex. First select which combination of spectral distrubtions to calculate. Then enter the frequency limits (in Hz) of the three contiguos bins that will define the spectral distribution.
      mask DialogControl ParameterGroupVar_copy Prompt: Spectral Distributions to Calculate
      mask DialogControl Control4 Prompt: Select which spectral distributions to calculate.
      mask DialogControl ParameterGroupVar Prompt: Bin Frequency Bands
      mask DialogControl Control2 Prompt: Enter the frequency limits (in Hz) inside square brackets for three contiguous bins (e.g. [5 10], [10 40], and [40 120]).
  Variance : Subsystem
  out_metrics : Outport
  wires:
  in_scg_sig/1 -> Average S2 peak-to-peak Amplitude Calculator/2(in_scg_signal), Average S1 peak-to-peak Amplitude Calculator/2(in_scg_sig), Spectral Distribution Calculator/2(in_scg_signal), Average Cycle-to-cycle Morphological Variability Calculator/2(in_scg_signal), Variance/1(in_scg_signal), Average Signal-to-Noise Ratio Calculator/2(in_scg_signal)
  Average S1 peak-to-peak Amplitude Calculator/1(out_average_s1p2pamp) -> Mux/1
  in_ecg_r_pos/1 -> Spectral Distribution Calculator/1(in_r_pos), Average Cycle-to-cycle Morphological Variability Calculator/1(in_r_pos), Average S2 peak-to-peak Amplitude Calculator/1(in_r_pos), Average S1 peak-to-peak Amplitude Calculator/1(in_r_pos), Average Signal-to-Noise Ratio Calculator/1(in_r_pos)
  Average Signal-to-Noise Ratio Calculator/2(out_scg_signal_average_s1Xsnr) -> Mux/4
  Average Signal-to-Noise Ratio Calculator/1(out_scg_signal_average_s1snr) -> Mux/3
  Average Signal-to-Noise Ratio Calculator/3(out_scg_signal_average_s2snr) -> Mux/5
  Average Signal-to-Noise Ratio Calculator/4(out_scg_signal_average_s2Xsnr) -> Mux/6
  Average S2 peak-to-peak Amplitude Calculator/1(out_scg_signal_average_s2p2pamp) -> Mux/2
  Average Cycle-to-cycle Morphological Variability Calculator/1(out_morphological_variability) -> Mux/8
  Spectral Distribution Calculator/1(out_entire_cycle_spectral_distribution) -> Mux/9
  Spectral Distribution Calculator/3(out_s2_spectral_distribution) -> Mux/11
  Spectral Distribution Calculator/2(out_s1_spectral_distribution) -> Mux/10
  Variance/1(out_scg_signal_var) -> Mux/7
  Constant/1 -> Average S1 peak-to-peak Amplitude Calculator/Enable
  Constant1/1 -> Average S2 peak-to-peak Amplitude Calculator/Enable
  Constant2/1 -> Average Signal-to-Noise Ratio Calculator/Enable
  Constant3/1 -> Variance/Enable
  Constant4/1 -> Average Cycle-to-cycle Morphological Variability Calculator/Enable
  Constant5/1 -> Spectral Distribution Calculator/Enable
  Mux/1 -> Display/1, out_metrics/1

== system FullCardioLablModel/SCG Analysis/Enabled SCG Analysis Subsystem/All Signals Signal Metric Characterization/SCG Systolic 3DMaxS1p2pProjection Signal Metric Characterization ==
  note: Spectral Distribution: S2 (Mid)
  note: Spectral Distribution: S2 (Lo)
  note: Spectral Distribution: S2 (Hi)
  note: Spectral Distribution: S1 (Hi)
  note: Spectral Distribution: S1 (Mid)
  note: Spectral Distribution: S1 (Lo)
  note: Spectral Distribution: Entire Cycle (Hi)
  note: Spectral Distribution: Entire Cycle (Mid)
  note: Spectral Distribution: Entire Cycle (Lo)
  note: Morphological Variability
  note: Var
  note: S2X SNR
  note: S2 SNR
  note: S1X SNR
  note: S1 SNR
  note: S2 P2P Amplitude
  note: S1 P2P Amplitude
  in_ecg_r_pos : Inport
  in_scg_sig : Inport  Port=2
  Average Cycle-to-cycle Morphological Variability Calculator : Subsystem
  Average S1 peak-to-peak Amplitude Calculator : Subsystem
  Average S2 peak-to-peak Amplitude Calculator : Subsystem
  Average Signal-to-Noise Ratio Calculator : Subsystem  mask{s1snr_flag=on, s1xsnr_flag=on, s2snr_flag=on, s2xsnr_flag=on}
      mask prompts: s1snr_flag "S1 SnR"; s1xsnr_flag "S1X SnR (S2 complex is removed)"; s2snr_flag "S2 SnR"; s2xsnr_flag "S2X SnR (S1 complex is removed)"
      mask DialogControl DescGroupVar Prompt: Signal-to-Noise Ratio Characterization
      mask DialogControl DescTextVar Prompt: Block to quantify the signal to noise ratio of the S1 and S2 complexes. Two types of SnRs can be calculated: the normal SnR (which reflects the ease of performing an independent detection of that complex), and the exclusive SnR (which does not cosider the S2 or S1 complex in the case of the S1 and S2 SnRs, respectively).
      mask DialogControl Control2 Prompt: Choose which SnRs to compute:
  Constant : Constant  Value=s1p2p_flag
  Constant1 : Constant  Value=s2p2p_flag
  Constant2 : Constant  Value=snr_flag
  Constant3 : Constant  Value=var_flag
  Constant4 : Constant  Value=morphvar_flag
  Constant5 : Constant  Value=nsd_flag
  Display : Display
  Mux : Mux  Inputs=11
  Spectral Distribution Calculator : Subsystem  mask{entire_cycle=on, s1=on, s2=on, f_band_lo=[7.5 15], f_band_mid=[15 30], f_band_hi=[30 120]}
      mask prompts: entire_cycle "Entire Cycle"; s1 "S1 Complex"; s2 "S2 Complex"; f_band_lo "Frequency Band Low Limits (Hz)"; f_band_mid "Frequency Band Mid Limits (Hz)"; f_band_hi "Frequency Band Hi Limits (Hz)"
      mask DialogControl DescGroupVar Prompt: Spectral Distribution Calculator
      mask DialogControl DescTextVar Prompt: Block to calculate the (normalized) distrubtions of the power spectral densities of: the entire cycle, the S1 complex, and the S2 complex. First select which combination of spectral distrubtions to calculate. Then enter the frequency limits (in Hz) of the three contiguos bins that will define the spectral distribution.
      mask DialogControl ParameterGroupVar_copy Prompt: Spectral Distributions to Calculate
      mask DialogControl Control4 Prompt: Select which spectral distributions to calculate.
      mask DialogControl ParameterGroupVar Prompt: Bin Frequency Bands
      mask DialogControl Control2 Prompt: Enter the frequency limits (in Hz) inside square brackets for three contiguous bins (e.g. [5 10], [10 40], and [40 120]).
  Variance : Subsystem
  out_metrics : Outport
  wires:
  Mux/1 -> out_metrics/1, Display/1
  Constant5/1 -> Spectral Distribution Calculator/Enable
  Constant4/1 -> Average Cycle-to-cycle Morphological Variability Calculator/Enable
  Constant3/1 -> Variance/Enable
  Constant2/1 -> Average Signal-to-Noise Ratio Calculator/Enable
  Constant1/1 -> Average S2 peak-to-peak Amplitude Calculator/Enable
  Constant/1 -> Average S1 peak-to-peak Amplitude Calculator/Enable
  Variance/1(out_scg_signal_var) -> Mux/7
  Spectral Distribution Calculator/2(out_s1_spectral_distribution) -> Mux/10
  Spectral Distribution Calculator/3(out_s2_spectral_distribution) -> Mux/11
  Spectral Distribution Calculator/1(out_entire_cycle_spectral_distribution) -> Mux/9
  Average Cycle-to-cycle Morphological Variability Calculator/1(out_morphological_variability) -> Mux/8
  Average S2 peak-to-peak Amplitude Calculator/1(out_scg_signal_average_s2p2pamp) -> Mux/2
  Average Signal-to-Noise Ratio Calculator/4(out_scg_signal_average_s2Xsnr) -> Mux/6
  Average Signal-to-Noise Ratio Calculator/3(out_scg_signal_average_s2snr) -> Mux/5
  Average Signal-to-Noise Ratio Calculator/1(out_scg_signal_average_s1snr) -> Mux/3
  Average Signal-to-Noise Ratio Calculator/2(out_scg_signal_average_s1Xsnr) -> Mux/4
  in_ecg_r_pos/1 -> Average Signal-to-Noise Ratio Calculator/1(in_r_pos), Average S1 peak-to-peak Amplitude Calculator/1(in_r_pos), Average S2 peak-to-peak Amplitude Calculator/1(in_r_pos), Average Cycle-to-cycle Morphological Variability Calculator/1(in_r_pos), Spectral Distribution Calculator/1(in_r_pos)
  Average S1 peak-to-peak Amplitude Calculator/1(out_average_s1p2pamp) -> Mux/1
  in_scg_sig/1 -> Average S1 peak-to-peak Amplitude Calculator/2(in_scg_sig), Average S2 peak-to-peak Amplitude Calculator/2(in_scg_signal), Average Signal-to-Noise Ratio Calculator/2(in_scg_signal), Variance/1(in_scg_signal), Average Cycle-to-cycle Morphological Variability Calculator/2(in_scg_signal), Spectral Distribution Calculator/2(in_scg_signal)
